simulink model "Punto2b_polo_extra"  (Simulink 7.5)
settings: Solver=ode45  StartTime=0  StopTime=3  MaxStep=0.001  RelTol=1e-3
settings Model: Creator=Nahuek  LastModifiedBy=Nahuek

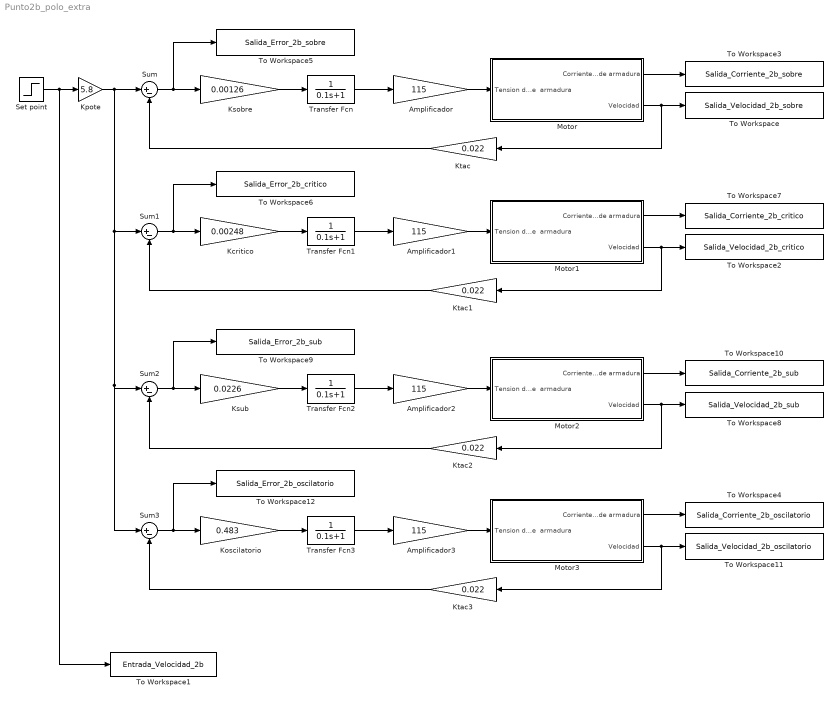
== system Punto2b_polo_extra ==
  Amplificador{,1..3} (4 alike) : Gain  Gain=115  ParameterDataType=fixdt(1, 16)  ParameterScaling=2^0  OutDataType=fixdt(1, 16)  OutScaling=2^0
  Kcritico : Gain  Gain=0.00248  ParameterDataType=fixdt(1, 16)  ParameterScaling=2^0  OutDataType=fixdt(1, 16)  OutScaling=2^0
  Koscilatorio : Gain  Gain=0.483  ParameterDataType=fixdt(1, 16)  ParameterScaling=2^0  OutDataType=fixdt(1, 16)  OutScaling=2^0
  Kpote : Gain  Gain=5.8  ParameterDataType=fixdt(1, 16)  ParameterScaling=2^0  OutDataType=fixdt(1, 16)  OutScaling=2^0
  Ksobre : Gain  Gain=0.00126  ParameterDataType=fixdt(1, 16)  ParameterScaling=2^0  OutDataType=fixdt(1, 16)  OutScaling=2^0
  Ksub : Gain  Gain=0.0226  ParameterDataType=fixdt(1, 16)  ParameterScaling=2^0  OutDataType=fixdt(1, 16)  OutScaling=2^0
  Ktac{,1..3} (4 alike) : Gain  Gain=0.022  ParameterDataType=fixdt(1, 16)  ParameterScaling=2^0  OutDataType=fixdt(1, 16)  OutScaling=2^0
  Motor : Subsystem
  Motor1 : Subsystem
  Motor2 : Subsystem
  Motor3 : Subsystem
  Set point : Step  Time=0  SampleTime=0
  Sum{,1..3} (4 alike) : Sum  Inputs=|+-  OutDataType=fixdt(1, 16)  OutScaling=2^0
  To Workspace : ToWorkspace  VariableName=Salida_Velocidad_2b_sobre  SampleTime=-1  SaveFormat=Structure With Time
  To Workspace1 : ToWorkspace  VariableName=Entrada_Velocidad_2b  SampleTime=-1  SaveFormat=Structure With Time
  To Workspace10 : ToWorkspace  VariableName=Salida_Corriente_2b_sub  SampleTime=-1  SaveFormat=Structure With Time
  To Workspace11 : ToWorkspace  VariableName=Salida_Velocidad_2b_oscilatorio  SampleTime=-1  SaveFormat=Structure With Time
  To Workspace12 : ToWorkspace  VariableName=Salida_Error_2b_oscilatorio  SampleTime=-1  SaveFormat=Structure With Time
  To Workspace2 : ToWorkspace  VariableName=Salida_Velocidad_2b_critico  SampleTime=-1  SaveFormat=Structure With Time
  To Workspace3 : ToWorkspace  VariableName=Salida_Corriente_2b_sobre  SampleTime=-1  SaveFormat=Structure With Time
  To Workspace4 : ToWorkspace  VariableName=Salida_Corriente_2b_oscilatorio  SampleTime=-1  SaveFormat=Structure With Time
  To Workspace5 : ToWorkspace  VariableName=Salida_Error_2b_sobre  SampleTime=-1  SaveFormat=Structure With Time
  To Workspace6 : ToWorkspace  VariableName=Salida_Error_2b_critico  SampleTime=-1  SaveFormat=Structure With Time
  To Workspace7 : ToWorkspace  VariableName=Salida_Corriente_2b_critico  SampleTime=-1  SaveFormat=Structure With Time
  To Workspace8 : ToWorkspace  VariableName=Salida_Velocidad_2b_sub  SampleTime=-1  SaveFormat=Structure With Time
  To Workspace9 : ToWorkspace  VariableName=Salida_Error_2b_sub  SampleTime=-1  SaveFormat=Structure With Time
  Transfer Fcn{,1..3} (4 alike) : TransferFcn  Denominator=[0.1 1]
  wires:
  Sum/1 -> Ksobre/1, To Workspace5/1
  Amplificador/1 -> Motor/1(Tension de  armadura)
  Motor/2(Velocidad) -> To Workspace/1, Ktac/1
  Ktac/1 -> Sum/2
  Kpote/1 -> Sum/1, Sum1/1, Sum2/1, Sum3/1
  Set point/1 -> Kpote/1, To Workspace1/1
  Motor/1(Corriente de armadura) -> To Workspace3/1
  Sum1/1 -> Kcritico/1, To Workspace6/1
  Amplificador1/1 -> Motor1/1(Tension de  armadura)
  Motor1/2(Velocidad) -> Ktac1/1, To Workspace2/1
  Ktac1/1 -> Sum1/2
  Motor1/1(Corriente de armadura) -> To Workspace7/1
  Sum2/1 -> Ksub/1, To Workspace9/1
  Amplificador2/1 -> Motor2/1(Tension de  armadura)
  Motor2/2(Velocidad) -> Ktac2/1, To Workspace8/1
  Ktac2/1 -> Sum2/2
  Motor2/1(Corriente de armadura) -> To Workspace10/1
  Transfer Fcn/1 -> Amplificador/1
  Ksobre/1 -> Transfer Fcn/1
  Transfer Fcn1/1 -> Amplificador1/1
  Kcritico/1 -> Transfer Fcn1/1
  Transfer Fcn2/1 -> Amplificador2/1
  Ksub/1 -> Transfer Fcn2/1
  Sum3/1 -> Koscilatorio/1, To Workspace12/1
  Amplificador3/1 -> Motor3/1(Tension de  armadura)
  Motor3/2(Velocidad) -> Ktac3/1, To Workspace11/1
  Ktac3/1 -> Sum3/2
  Motor3/1(Corriente de armadura) -> To Workspace4/1
  Transfer Fcn3/1 -> Amplificador3/1
  Koscilatorio/1 -> Transfer Fcn3/1

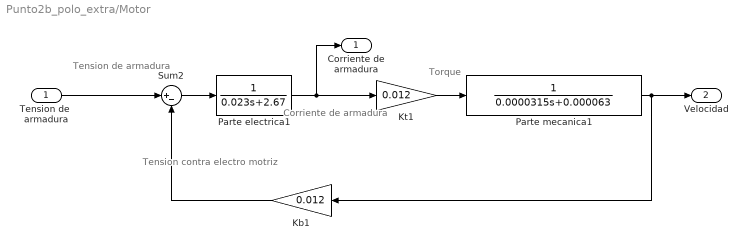
== system Punto2b_polo_extra/Motor ==
  note: Tension contra
      |  electro motriz
  note: Corriente de
      | armadura
  note: Torque
  note: Tension de
      |  armadura
  Tension de  armadura : Inport
  Kb1 : Gain  Gain=0.012  ParameterDataType=fixdt(1, 16)  ParameterScaling=2^0  OutDataType=fixdt(1, 16)  OutScaling=2^0
  Kt1 : Gain  Gain=0.012  ParameterDataType=fixdt(1, 16)  ParameterScaling=2^0  OutDataType=fixdt(1, 16)  OutScaling=2^0
  Parte electrica1 : TransferFcn  Denominator=[0.023 2.67]
  Parte mecanica1 : TransferFcn  Denominator=[0.0000315 0.000063]
  Sum2 : Sum  Inputs=|+-  OutDataType=fixdt(1, 16)  OutScaling=2^0
  Corriente de armadura : Outport
  Velocidad : Outport  Port=2
  wires:
  Sum2/1 -> Parte electrica1/1
  Kt1/1 -> Parte mecanica1/1
  Parte electrica1/1 -> Kt1/1, Corriente de armadura/1
  Kb1/1 -> Sum2/2
  Parte mecanica1/1 -> Kb1/1, Velocidad/1
  Tension de  armadura/1 -> Sum2/1

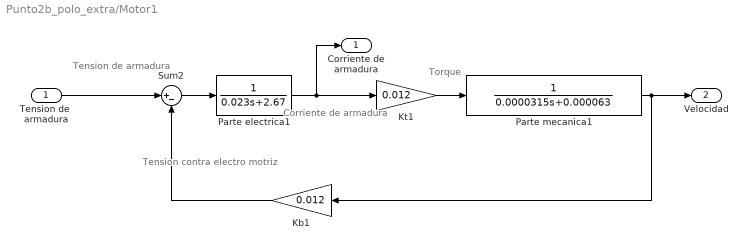
== system Punto2b_polo_extra/Motor1 ==
  note: Tension contra
      |  electro motriz
  note: Corriente de
      | armadura
  note: Torque
  note: Tension de
      |  armadura
  Tension de  armadura : Inport
  Kb1 : Gain  Gain=0.012  ParameterDataType=fixdt(1, 16)  ParameterScaling=2^0  OutDataType=fixdt(1, 16)  OutScaling=2^0
  Kt1 : Gain  Gain=0.012  ParameterDataType=fixdt(1, 16)  ParameterScaling=2^0  OutDataType=fixdt(1, 16)  OutScaling=2^0
  Parte electrica1 : TransferFcn  Denominator=[0.023 2.67]
  Parte mecanica1 : TransferFcn  Denominator=[0.0000315 0.000063]
  Sum2 : Sum  Inputs=|+-  OutDataType=fixdt(1, 16)  OutScaling=2^0
  Corriente de armadura : Outport
  Velocidad : Outport  Port=2
  wires:
  Sum2/1 -> Parte electrica1/1
  Kt1/1 -> Parte mecanica1/1
  Parte electrica1/1 -> Kt1/1, Corriente de armadura/1
  Kb1/1 -> Sum2/2
  Parte mecanica1/1 -> Kb1/1, Velocidad/1
  Tension de  armadura/1 -> Sum2/1

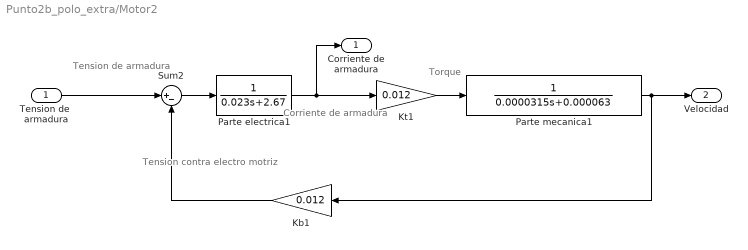
== system Punto2b_polo_extra/Motor2 ==
  note: Tension contra
      |  electro motriz
  note: Corriente de
      | armadura
  note: Torque
  note: Tension de
      |  armadura
  Tension de  armadura : Inport
  Kb1 : Gain  Gain=0.012  ParameterDataType=fixdt(1, 16)  ParameterScaling=2^0  OutDataType=fixdt(1, 16)  OutScaling=2^0
  Kt1 : Gain  Gain=0.012  ParameterDataType=fixdt(1, 16)  ParameterScaling=2^0  OutDataType=fixdt(1, 16)  OutScaling=2^0
  Parte electrica1 : TransferFcn  Denominator=[0.023 2.67]
  Parte mecanica1 : TransferFcn  Denominator=[0.0000315 0.000063]
  Sum2 : Sum  Inputs=|+-  OutDataType=fixdt(1, 16)  OutScaling=2^0
  Corriente de armadura : Outport
  Velocidad : Outport  Port=2
  wires:
  Sum2/1 -> Parte electrica1/1
  Kt1/1 -> Parte mecanica1/1
  Parte electrica1/1 -> Kt1/1, Corriente de armadura/1
  Kb1/1 -> Sum2/2
  Parte mecanica1/1 -> Kb1/1, Velocidad/1
  Tension de  armadura/1 -> Sum2/1

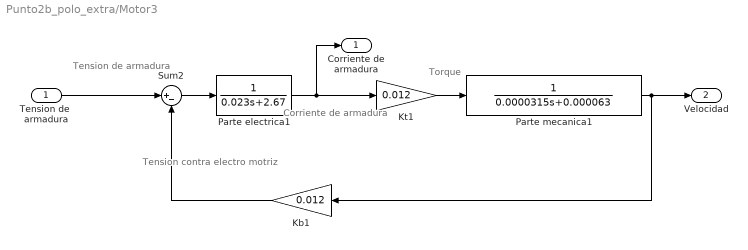
== system Punto2b_polo_extra/Motor3 ==
  note: Tension contra
      |  electro motriz
  note: Corriente de
      | armadura
  note: Torque
  note: Tension de
      |  armadura
  Tension de  armadura : Inport
  Kb1 : Gain  Gain=0.012  ParameterDataType=fixdt(1, 16)  ParameterScaling=2^0  OutDataType=fixdt(1, 16)  OutScaling=2^0
  Kt1 : Gain  Gain=0.012  ParameterDataType=fixdt(1, 16)  ParameterScaling=2^0  OutDataType=fixdt(1, 16)  OutScaling=2^0
  Parte electrica1 : TransferFcn  Denominator=[0.023 2.67]
  Parte mecanica1 : TransferFcn  Denominator=[0.0000315 0.000063]
  Sum2 : Sum  Inputs=|+-  OutDataType=fixdt(1, 16)  OutScaling=2^0
  Corriente de armadura : Outport
  Velocidad : Outport  Port=2
  wires:
  Sum2/1 -> Parte electrica1/1
  Kt1/1 -> Parte mecanica1/1
  Parte electrica1/1 -> Kt1/1, Corriente de armadura/1
  Kb1/1 -> Sum2/2
  Parte mecanica1/1 -> Kb1/1, Velocidad/1
  Tension de  armadura/1 -> Sum2/1
